simulink model "Planta1"  (R2026a)
settings: Solver=ode4  FixedStep=1e-4
settings Model: Creator=Yahoff  LastModifiedBy=Yahoff

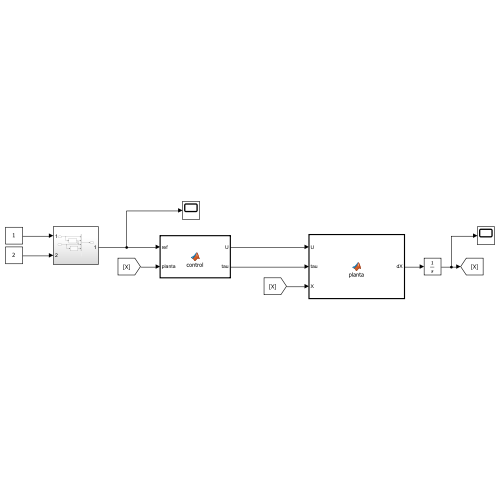
[thumbnail: Simulink's stored preview of the top-level diagram]
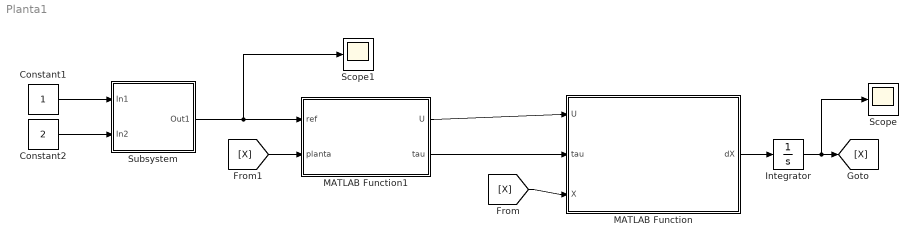
== system Planta1 ==
  Constant1 : Constant
  Constant2 : Constant  Value=2
  Integrator : Integrator  InitialCondition=[0;0;0;0;0;0]
  MATLAB Function : MATLAB Function  TreatAsAtomicUnit=on
  MATLAB Function1 : MATLAB Function  TreatAsAtomicUnit=on
  Scope : Scope
      settings: ActiveDisplayYMinimum=-2.707620287076792E+22  ActiveDisplayYMaximum=5.7996413011817377E+22
  Scope1 : Scope
      settings: ActiveDisplayYMinimum=-1  ActiveDisplayYMaximum=1
  Subsystem : Subsystem
  wires:
  MATLAB Function/1(dX) -> Integrator/1
  Integrator/1 -> Scope/1, [X]
  [X] -> MATLAB Function/3(X)
  [X] -> MATLAB Function1/2(planta)
  MATLAB Function1/1(U) -> MATLAB Function/1(U)
  MATLAB Function1/2(tau) -> MATLAB Function/2(tau)
  Subsystem/1(Out1) -> Scope1/1, MATLAB Function1/1(ref)
  Constant1/1 -> Subsystem/1(In1)
  Constant2/1 -> Subsystem/2(In2)

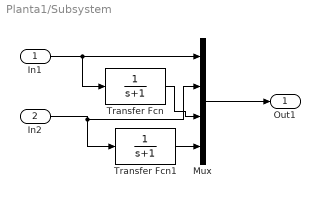
== system Planta1/Subsystem ==
  In1 : Inport
  In2 : Inport  Port=2
  Mux : Mux
  Transfer Fcn : TransferFcn  Denominator=[1 1]
  Transfer Fcn1 : TransferFcn  Denominator=[1 1]
  Out1 : Outport
  wires:
  Transfer Fcn/1 -> Mux/3
  Transfer Fcn1/1 -> Mux/4
  In1/1 -> Transfer Fcn/1, Mux/1
  Mux/1 -> Out1/1
  In2/1 -> Mux/2, Transfer Fcn1/1

== matlab function Planta1/MATLAB Function ==
  data: U input; dX output; tau input; X input
function dX = planta(U, tau, X)

    m = 1; J = 1; g = 9.81;

    x     = X(1);
    xdot  = X(2);
    z     = X(3);
    zdot  = X(4);
    th    = X(5);
    thdot = X(6);

    xdd  = -(U/m)*sin(th);
    zdd  =  (U/m)*cos(th) - g;
    thdd =  tau/J;

    dX = [xdot; xdd; zdot; zdd; thdot; thdd];

== matlab function Planta1/MATLAB Function1 ==
  data: ref input; U output; planta input; tau output
function [U, tau] = control(ref, planta)

    m = 1; g = 9.81;
    kp = 4;  kd = 4;
    kth = 30; kom = 12;

    xr = ref(1);
    zr = ref(2);
    ux = ref(3);   
    uz = ref(4);   

    x     = planta(1);
    xdot  = planta(2);
    z     = planta(3);
    zdot  = planta(4);
    th    = planta(5);
    thdot = planta(6);

    xrd  = ux - xr;    xrdd = -(ux - xr);
    zrd  = uz - zr;    zrdd = -(uz - zr);

    vx = xrdd - kp*(x - xr) - kd*(xdot - xrd);
    vz = zrdd - kp*(z - zr) - kd*(zdot - zrd);

    U   = m*sqrt(vx^2 + (vz+g)^2);
    thd = atan2(-vx, vz+g);

    tau = -kth*(th - thd) - kom*thdot;
end
